simulink model "for_fft_dif"  (R2018a)
settings: Solver=FixedStepAuto  StartTime=0.0  StopTime=time_array2(end)  FixedStep=Tstep  RelTol=1e-3  EnableMultiTasking=on
values from neighbouring files (symbols this model uses):
  Tstep = time_array(2) - time_array(1)    [parallel_dif_unbalance_fft_analizleri.m]    (also in parallel_fft_analizleri.m; parallel_unbalance_fft_analizleri.m)
libraries: powerlib x1
settings Model: Creator=mesutto  LastModifiedBy=gizemlikaradenizli61
settings OptimizationCC: LifeSpan=inf
settings DebuggingCC: SFUnexpectedBacktrackingDiag=warning  SFNoUnconditionalDefaultTransitionDiag=warning  SFExecutionAtInitializationDiag=none
settings CodeAppCC: StateflowObjectComments=on
settings GRTTargetCC: TargetLangStandard=C89/C90 (ANSI)  GeneratePreprocessorConditionals=Disable all
settings ConfigComp: CovMetricSettings=dw  CovHtmlReporting=on  CovSaveCumulativeToWorkspaceVar=on  CovSaveSingleToWorkspaceVar=on  CovExternalEMLEnable=off

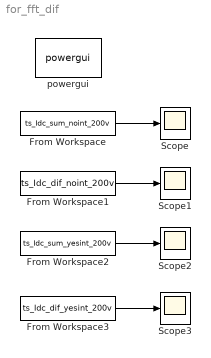
== system for_fft_dif ==
  From Workspace : FromWorkspace  VariableName=ts_Idc_sum_noint_200v  SampleTime=Tstep
  From Workspace1 : FromWorkspace  VariableName=ts_Idc_dif_noint_200v  SampleTime=Tstep
  From Workspace2 : FromWorkspace  VariableName=ts_Idc_sum_yesint_200v  SampleTime=Tstep
  From Workspace3 : FromWorkspace  VariableName=ts_Idc_dif_yesint_200v  SampleTime=Tstep
  Scope{,1..3} (4 alike) : Scope
  powergui : powerlib/powergui  Priority=1  SimulationMode=Discrete  SampleTime=Tstep  frequency=60  Iterations=50  frequencyindice=60  Pbase=100e6  ErrMax=1e-4  UnitsV=kV  UnitsW=MW  buscounter=0  FunctionMessages=off  echomessages=off  EnableUseOfTLC=off  CurrentSourceSwitches=off  DisableSnubberDevices=off  DisableRonSwitches=off  DisableVfSwitches=off  DisplayEquations=off  SolverType=Tustin/Backward Euler (TBE)  Interpol=off  ExternalGateDelay=off  methode=off  Ts=100  x0status=blocks  SPID=off  SwTol=0  HookPort=off  RestoreLinks=warning  ResistiveCurrentMeasurement=off  Frange=[0:2:500]  Ylog=off  Xlog=on  ShowGrid=off  save=off  variable=ZData  structure=0  ZoomFFT=off  StartTime=0.0  cycles=1  DisplayStyle=1  fundamental=60  FreqAxis=off  MaxFrequency=1000  frequencyindicesteady=1  RmsSteady=1  display=off
  wires:
  From Workspace/1 -> Scope/1
  From Workspace1/1 -> Scope1/1
  From Workspace2/1 -> Scope2/1
  From Workspace3/1 -> Scope3/1
